simulink model "Problem5"  (R2020b)
settings: Solver=VariableStepAuto  StartTime=0.0  StopTime=10.0  RelTol=1e-3
model workspace (MAT data in the model file):
  C = 1e-07
  R = 10
  q = 5
settings Model: Creator=Dell  LastModifiedBy=DELL

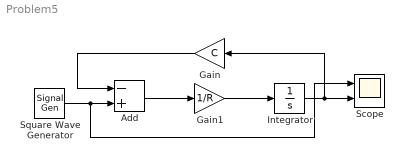
== system Problem5 ==
  Add : Sum  Inputs=-+
  Gain : Gain  Gain=C
  Gain1 : Gain  Gain=1/R
  Integrator : Integrator
  Scope : Scope  NumInputPorts=2
  Square Wave Generator : SignalGenerator  WaveForm=square  Units=rad/sec
  wires:
  Square Wave Generator/1 -> Scope/1, Add/2
  Gain/1 -> Add/1
  Add/1 -> Gain1/1
  Gain1/1 -> Integrator/1
  Integrator/1 -> Gain/1, Scope/2
